simulink model "kalmanfilter"  (R2024b)
settings: Solver=FixedStepAuto  StartTime=0.0  StopTime=10.0  FixedStep=1  RelTol=1e-3
settings Model: Creator=54238  LastModifiedBy=54238

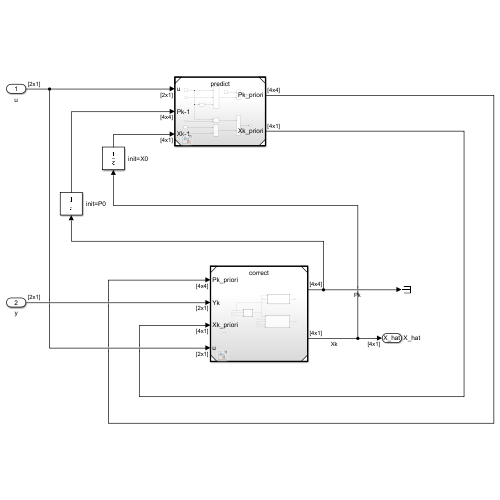
[thumbnail: Simulink's stored preview of the top-level diagram]
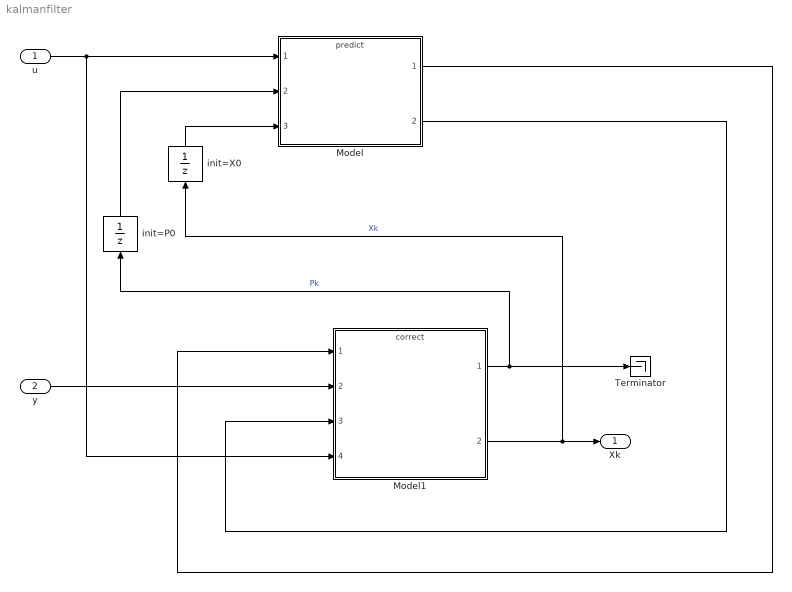
== system kalmanfilter ==
  u : Inport  PortDimensions=[2,1]
  y : Inport  Port=2  PortDimensions=[2,1]
  Model : ModelReference  ModelNameDialog=predict.slx  SimulationMode=Normal  ModelReferenceVersion=1.6
  Model1 : ModelReference  ModelNameDialog=correct.slx  SimulationMode=Normal  ModelReferenceVersion=1.6
  Terminator : Terminator
  init=P0 : UnitDelay  SampleTime=-1  StateName=p0  HasFrameUpgradeWarning=on
  init=X0 : UnitDelay  SampleTime=-1  HasFrameUpgradeWarning=on
  Xk : Outport  SignalName=X_hat  PortDimensions=[4,1]
  wires:
  u/1 -> Model1/4, Model/1
  init=P0/1 -> Model/2
  init=X0/1 -> Model/3
  y/1 -> Model1/2
  Model1/1 -> init=P0/1, Terminator/1  "Pk"
  Model1/2 -> Xk/1, init=X0/1  "Xk"
  Model/1 -> Model1/1
  Model/2 -> Model1/3
